simulink model "gm_uz_JL_pmsmModel"  (R2025a)
settings: Solver=FixedStepDiscrete  StartTime=0.0  StopTime=1  RelTol=1e-3
libraries: hdlmdlgenlib x2
(part 1 of 2)
settings Model: Creator=jonat  LastModifiedBy=jonat
settings SolverCC: AlgebraicLoopSolver=TrustRegion
settings DataIOCC: LimitDataPoints=on  SaveOutput=off  SaveTime=off
settings OptimizationCC: BlockReduction=off  ConditionallyExecuteInputs=off  DefaultParameterBehavior=Inlined  InheritOutputTypeSmallerThanSingle=on  DefaultUnderspecifiedDataType=single  LifeSpan=inf
settings DebuggingCC: AlgebraicLoopMsg=error  InheritedTsInSrcMsg=none  SingleTaskRateTransMsg=error  SignalLabelMismatchMsg=warning  UnconnectedInputMsg=warning  UnconnectedOutputMsg=warning  UnconnectedLineMsg=warning  AllowSymbolicDim=off  ModelReferenceVersionMismatchMessage=warning  ModelReferenceIOMismatchMessage=warning  ModelReferenceNoExplicitFinalValueMsg=warning  StrictBusMsg=ErrorOnBusTreatedAsVector  BusNameAdapt=ErrorWithoutRepair  SFUnexpectedBacktrackingDiag=warning  SFNoUnconditionalDefaultTransitionDiag=warning  SFExecutionAtInitializationDiag=none  ArithmeticOperatorsInVariantConditions=warning
settings HardwareCC: ProdBitPerPointer=32.0  ProdBitPerSizeT=32.0  ProdBitPerPtrDiffT=32.0  ProdLargestAtomicFloat=None  ProdIntDivRoundTo=Undefined  ProdEndianess=Unspecified  ProdWordSize=32.0  ProdHWDeviceType=ASIC/FPGA->ASIC/FPGA  TargetBitPerPointer=64.0  TargetBitPerSizeT=64.0  TargetBitPerPtrDiffT=64.0  TargetLongLongMode=on  TargetIntDivRoundTo=Zero  TargetEndianess=LittleEndian  TargetWordSize=64.0  TargetHWDeviceType=Custom Processor->MATLAB Host Computer  ProdEqTarget=off
settings ModelReferenceCC: EnableRefExpFcnMdlSchedulingChecks=on
settings SFSimCC: SimUseLocalCustomCode=off  CustomCodeUndefinedFunction=UseInterfaceOnly
settings RTWCC: RTWUseLocalCustomCode=off  GPUComputeCapability=3.5
settings CodeAppCC: StateflowObjectComments=on
settings GRTTargetCC: TargetLangStandard=C89/C90 (ANSI)
settings ConfigComp: CovScope=ReferencedModels  CovMetricSettings=dw  CovSaveCumulativeToWorkspaceVar=on  CovSaveSingleToWorkspaceVar=on  CovExternalEMLEnable=off  CovSFcnEnable=off

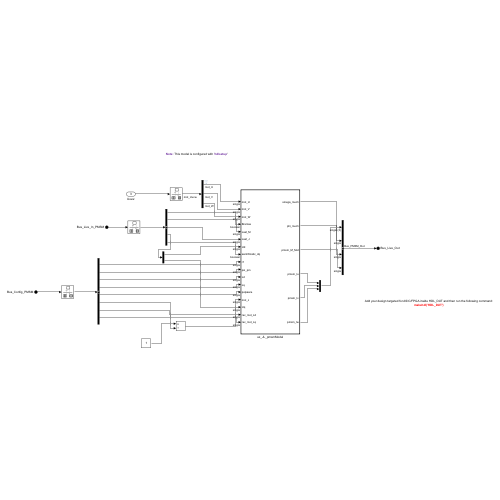
[thumbnail: Simulink's stored preview of the top-level diagram]
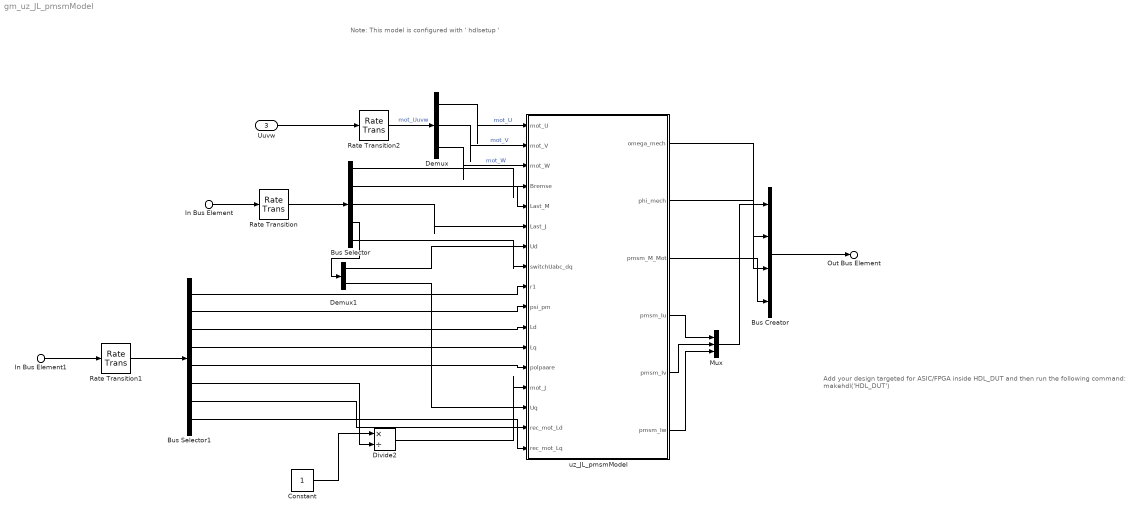
== system gm_uz_JL_pmsmModel ==
  note: Add your design targeted for ASIC/FPGA inside HDL_DUT and then run the following command:
      | makehdl('HDL_DUT')
  note: Note: This model is configured with ' hdlsetup '
  In Bus Element : Inport  PortName=Bus_Live_In_PMSM
  In Bus Element1 : Inport  Port=2  PortName=Bus_Config_PMSM
  Uuvw : Inport  Port=3
  Bus Creator : BusCreator  Inputs=4  OutDataTypeStr=Bus: Bus_PMSM_Out  NonVirtualBus=on
      settings: InheritFromInputs=off
  Bus Selector : BusSelector  OutputSignals=Bremse,Last_M,Last_J,Udq,switchUabc_dq
  Bus Selector1 : BusSelector  OutputSignals=mot_R1,mot_psi_pm,mot_Ld,mot_Lq,mot_p,mot_J,rec_mot_Ld,rec_mot_Lq
  Constant : Constant
  Demux : Demux  Outputs=3
  Demux1 : Demux  Outputs=2
  Divide2 : Product  Inputs=*/  OutDataTypeStr=single
  Mux : Mux  Inputs=3
  Rate Transition : RateTransition  OutPortSampleTime=1/5e5
  Rate Transition1 : RateTransition  OutPortSampleTime=1/5e5
  Rate Transition2 : RateTransition  OutPortSampleTime=1/5e5
  uz_JL_pmsmModel : Subsystem  TreatAsAtomicUnit=on
  Out Bus Element : Outport  PortName=Bus_Live_Out
  wires:
  Bus Selector1/8 -> uz_JL_pmsmModel/17(rec_mot_Lq)
  Bus Selector1/7 -> uz_JL_pmsmModel/16(rec_mot_Ld)
  Demux1/2 -> uz_JL_pmsmModel/15(Uq)
  Demux1/1 -> uz_JL_pmsmModel/7(Ud)
  Mux/1 -> Bus Creator/1
  uz_JL_pmsmModel/6(pmsm_Iw) -> Mux/3
  uz_JL_pmsmModel/5(pmsm_Iv) -> Mux/2
  uz_JL_pmsmModel/4(pmsm_Iu) -> Mux/1
  Demux/1 -> uz_JL_pmsmModel/1(mot_U)  "mot_U"
  Rate Transition2/1 -> Demux/1  "mot_Uuvw"
  Demux/2 -> uz_JL_pmsmModel/2(mot_V)  "mot_V"
  Demux/3 -> uz_JL_pmsmModel/3(mot_W)  "mot_W"
  Divide2/1 -> uz_JL_pmsmModel/14(mot_J)
  Constant/1 -> Divide2/1
  uz_JL_pmsmModel/3(pmsm_M_Mot) -> Bus Creator/4
  uz_JL_pmsmModel/2(phi_mech) -> Bus Creator/3
  uz_JL_pmsmModel/1(omega_mech) -> Bus Creator/2
  Bus Selector1/6 -> Divide2/2
  Bus Selector1/5 -> uz_JL_pmsmModel/13(polpaare)
  Bus Selector1/4 -> uz_JL_pmsmModel/12(Lq)
  Bus Selector1/3 -> uz_JL_pmsmModel/11(Ld)
  Bus Selector1/2 -> uz_JL_pmsmModel/10(psi_pm)
  Bus Selector1/1 -> uz_JL_pmsmModel/9(r1)
  Bus Selector/5 -> uz_JL_pmsmModel/8(switchUabc_dq)
  Bus Selector/4 -> Demux1/1
  Bus Selector/3 -> uz_JL_pmsmModel/6(Last_J)
  Bus Selector/2 -> uz_JL_pmsmModel/5(Last_M)
  Bus Selector/1 -> uz_JL_pmsmModel/4(Bremse)
  Uuvw/1 -> Rate Transition2/1
  Rate Transition1/1 -> Bus Selector1/1
  Rate Transition/1 -> Bus Selector/1
  Bus Creator/1 -> Out Bus Element/1
  In Bus Element1/1 -> Rate Transition1/1
  In Bus Element/1 -> Rate Transition/1

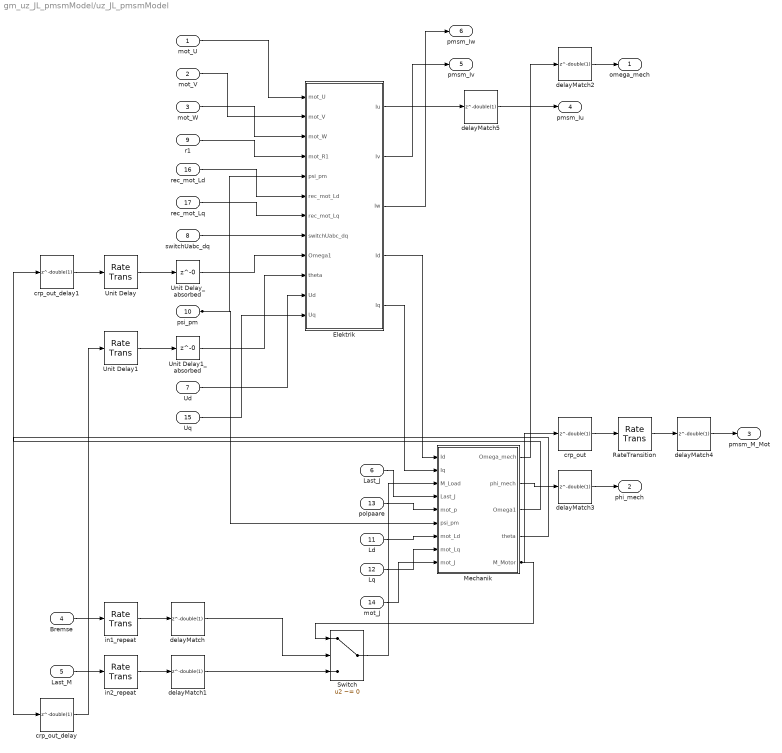
== system gm_uz_JL_pmsmModel/uz_JL_pmsmModel ==
  mot_U : Inport  OutDataTypeStr=single  PortDimensions=1  SampleTime=2e-06
  mot_V : Inport  Port=2  OutDataTypeStr=single  PortDimensions=1  SampleTime=2e-06
  mot_W : Inport  Port=3  OutDataTypeStr=single  PortDimensions=1  SampleTime=2e-06
  Bremse : Inport  Port=4  OutDataTypeStr=boolean  PortDimensions=1  SampleTime=2e-06
  Last_M : Inport  Port=5  OutDataTypeStr=single  PortDimensions=1  SampleTime=2e-06
  Last_J : Inport  Port=6  OutDataTypeStr=single  PortDimensions=1  SampleTime=2e-06
  Ud : Inport  Port=7  OutDataTypeStr=single  PortDimensions=1  SampleTime=2e-06
  switchUabc_dq : Inport  Port=8  OutDataTypeStr=boolean  PortDimensions=1  SampleTime=2e-06
  r1 : Inport  Port=9  OutDataTypeStr=single  PortDimensions=1  SampleTime=2e-06
  psi_pm : Inport  Port=10  OutDataTypeStr=single  PortDimensions=1  SampleTime=2e-06
  Ld : Inport  Port=11  OutDataTypeStr=single  PortDimensions=1  SampleTime=2e-06
  Lq : Inport  Port=12  OutDataTypeStr=single  PortDimensions=1  SampleTime=2e-06
  polpaare : Inport  Port=13  OutDataTypeStr=single  PortDimensions=1  SampleTime=2e-06
  mot_J : Inport  Port=14  OutDataTypeStr=single  PortDimensions=1  SampleTime=2e-06
  Uq : Inport  Port=15  OutDataTypeStr=single  PortDimensions=1  SampleTime=2e-06
  rec_mot_Ld : Inport  Port=16  OutDataTypeStr=single  PortDimensions=1  SampleTime=2e-06
  rec_mot_Lq : Inport  Port=17  OutDataTypeStr=single  PortDimensions=1  SampleTime=2e-06
  Elektrik : Subsystem
  Mechanik : Subsystem
  RateTransition : RateTransition  InitialCondition=double(0)  OutPortSampleTimeOpt=Multiple of input port sample time  OutPortSampleTimeMultiple=100
  Switch : Switch  Criteria=u2 ~= 0  Threshold="fi(0,0,1,0,\"hex\",\"0\")"  OutDataTypeStr=single  SampleTime=2e-08  SaturateOnIntegerOverflow=off  InputSameDT=off
  Unit Delay : RateTransition  InitialCondition=double(0)  OutPortSampleTimeOpt=Multiple of input port sample time  OutPortSampleTimeMultiple=100
  Unit Delay1 : RateTransition  InitialCondition=double(0)  OutPortSampleTimeOpt=Multiple of input port sample time  OutPortSampleTimeMultiple=100
  Unit Delay1_absorbed : Delay  DelayLength=0
  Unit Delay_absorbed : Delay  DelayLength=0
  crp_out : Delay  DelayLength=double(1)  InitialCondition=0  SampleTime=2e-08
  crp_out_delay : Delay  DelayLength=double(1)  InitialCondition=0  SampleTime=2e-08
  crp_out_delay1 : Delay  DelayLength=double(1)  InitialCondition=0  SampleTime=2e-08
  delayMatch : Delay  DelayLength=double(1)  InitialCondition=0  SampleTime=2e-08
  delayMatch1 : Delay  DelayLength=double(1)  InitialCondition=0  SampleTime=2e-08
  delayMatch{2..5} (4 alike) : Delay  DelayLength=double(1)  InitialCondition=0  SampleTime=2e-06
  in1_repeat : RateTransition  Integrity=off  Deterministic=off  OutPortSampleTimeOpt=Multiple of input port sample time  OutPortSampleTimeMultiple=1/100
  in2_repeat : RateTransition  Integrity=off  Deterministic=off  OutPortSampleTimeOpt=Multiple of input port sample time  OutPortSampleTimeMultiple=1/100
  omega_mech : Outport  SampleTime=2e-06
  phi_mech : Outport  Port=2  SampleTime=2e-06
  pmsm_M_Mot : Outport  Port=3  SampleTime=2e-06
  pmsm_Iu : Outport  Port=4  SampleTime=2e-06
  pmsm_Iv : Outport  Port=5  SampleTime=2e-06
  pmsm_Iw : Outport  Port=6  SampleTime=2e-06
  wires:
  in2_repeat/1 -> delayMatch1/1
  crp_out_delay1/1 -> Unit Delay/1
  Unit Delay/1 -> Unit Delay_absorbed/1
  Ud/1 -> Elektrik/11(Ud)
  Bremse/1 -> in1_repeat/1
  Unit Delay1/1 -> Unit Delay1_absorbed/1
  Last_M/1 -> in2_repeat/1
  crp_out_delay/1 -> Unit Delay1/1
  in1_repeat/1 -> delayMatch/1
  Elektrik/2(Iv) -> pmsm_Iv/1
  mot_U/1 -> Elektrik/1(mot_U)
  polpaare/1 -> Mechanik/5(mot_p)
  mot_V/1 -> Elektrik/2(mot_V)
  delayMatch/1 -> Switch/2
  mot_W/1 -> Elektrik/3(mot_W)
  delayMatch4/1 -> pmsm_M_Mot/1
  r1/1 -> Elektrik/4(mot_R1)
  Elektrik/5(Iq) -> Mechanik/2(Iq)
  rec_mot_Ld/1 -> Elektrik/6(rec_mot_Ld)
  rec_mot_Lq/1 -> Elektrik/7(rec_mot_Lq)
  Mechanik/3(Omega1) -> crp_out_delay1/1
  switchUabc_dq/1 -> Elektrik/8(switchUabc_dq)
  Unit Delay_absorbed/1 -> Elektrik/9(Omega1)
  psi_pm/1 -> Mechanik/6(psi_pm), Elektrik/5(psi_pm)
  Switch/1 -> Mechanik/3(M_Load)
  Unit Delay1_absorbed/1 -> Elektrik/10(theta)
  Uq/1 -> Elektrik/12(Uq)
  Ld/1 -> Mechanik/7(mot_Ld)
  Elektrik/4(Id) -> Mechanik/1(Id)
  delayMatch1/1 -> Switch/3
  Elektrik/1(Iu) -> delayMatch5/1
  Elektrik/3(Iw) -> pmsm_Iw/1
  Last_J/1 -> Mechanik/4(Last_J)
  Lq/1 -> Mechanik/8(mot_Lq)
  delayMatch3/1 -> phi_mech/1
  mot_J/1 -> Mechanik/9(mot_J)
  delayMatch5/1 -> pmsm_Iu/1
  Mechanik/1(Omega_mech) -> delayMatch2/1
  Mechanik/2(phi_mech) -> delayMatch3/1
  Mechanik/4(theta) -> crp_out_delay/1
  Mechanik/5(M_Motor) -> crp_out/1, Switch/1
  delayMatch2/1 -> omega_mech/1
  crp_out/1 -> RateTransition/1
  RateTransition/1 -> delayMatch4/1

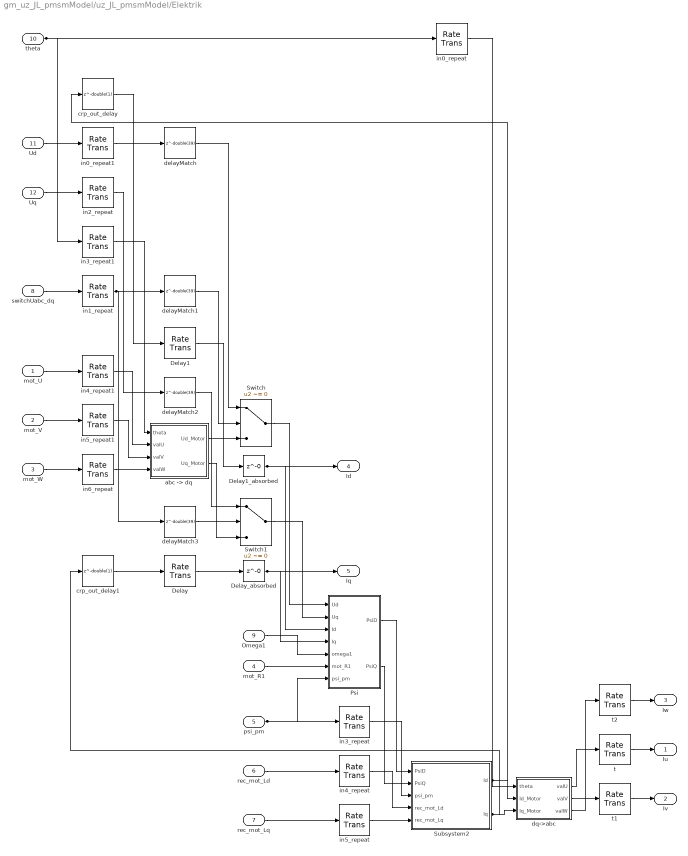
== system gm_uz_JL_pmsmModel/uz_JL_pmsmModel/Elektrik ==
  mot_U : Inport  OutDataTypeStr=single  PortDimensions=1  SampleTime=2e-06
  mot_V : Inport  Port=2  OutDataTypeStr=single  PortDimensions=1  SampleTime=2e-06
  mot_W : Inport  Port=3  OutDataTypeStr=single  PortDimensions=1  SampleTime=2e-06
  mot_R1 : Inport  Port=4  OutDataTypeStr=single  PortDimensions=1  SampleTime=2e-06
  psi_pm : Inport  Port=5  OutDataTypeStr=single  PortDimensions=1  SampleTime=2e-06
  rec_mot_Ld : Inport  Port=6  OutDataTypeStr=single  PortDimensions=1  SampleTime=2e-06
  rec_mot_Lq : Inport  Port=7  OutDataTypeStr=single  PortDimensions=1  SampleTime=2e-06
  switchUabc_dq : Inport  Port=8  OutDataTypeStr=boolean  PortDimensions=1  SampleTime=2e-06
  Omega1 : Inport  Port=9  OutDataTypeStr=single  PortDimensions=1  SampleTime=2e-06
  theta : Inport  Port=10  OutDataTypeStr=single  PortDimensions=1  SampleTime=2e-06
  Ud : Inport  Port=11  OutDataTypeStr=single  PortDimensions=1  SampleTime=2e-06
  Uq : Inport  Port=12  OutDataTypeStr=single  PortDimensions=1  SampleTime=2e-06
  Delay : RateTransition  InitialCondition=double(0)  OutPortSampleTimeOpt=Multiple of input port sample time  OutPortSampleTimeMultiple=100
  Delay1 : RateTransition  InitialCondition=double(0)  OutPortSampleTimeOpt=Multiple of input port sample time  OutPortSampleTimeMultiple=100
  Delay1_absorbed : Delay  DelayLength=0
  Delay_absorbed : Delay  DelayLength=0
  Psi : Subsystem
  Subsystem2 : Subsystem
  Switch : Switch  Criteria=u2 ~= 0  Threshold="fi(0,0,1,0,\"hex\",\"0\")"  OutDataTypeStr=single  SampleTime=2e-08  SaturateOnIntegerOverflow=off  InputSameDT=off
  Switch1 : Switch  Criteria=u2 ~= 0  Threshold="fi(0,0,1,0,\"hex\",\"0\")"  OutDataTypeStr=single  SampleTime=2e-08  SaturateOnIntegerOverflow=off  InputSameDT=off
  "abc -> dq" : Subsystem
  crp_out_delay : Delay  DelayLength=double(1)  InitialCondition=0  SampleTime=2e-08
  crp_out_delay1 : Delay  DelayLength=double(1)  InitialCondition=0  SampleTime=2e-08
  delayMatch{,1..3} (4 alike) : Delay  DelayLength=double(39)  InitialCondition=0  SampleTime=2e-08
  dq->abc : Subsystem
  in0_repeat : RateTransition  Integrity=off  Deterministic=off  OutPortSampleTimeOpt=Multiple of input port sample time  OutPortSampleTimeMultiple=1/100
  in0_repeat1 : RateTransition  Integrity=off  Deterministic=off  OutPortSampleTimeOpt=Multiple of input port sample time  OutPortSampleTimeMultiple=1/100
  in1_repeat : RateTransition  Integrity=off  Deterministic=off  OutPortSampleTimeOpt=Multiple of input port sample time  OutPortSampleTimeMultiple=1/100
  in2_repeat : RateTransition  Integrity=off  Deterministic=off  OutPortSampleTimeOpt=Multiple of input port sample time  OutPortSampleTimeMultiple=1/100
  in3_repeat : RateTransition  Integrity=off  Deterministic=off  OutPortSampleTimeOpt=Multiple of input port sample time  OutPortSampleTimeMultiple=1/100
  in3_repeat1 : RateTransition  Integrity=off  Deterministic=off  OutPortSampleTimeOpt=Multiple of input port sample time  OutPortSampleTimeMultiple=1/100
  in4_repeat : RateTransition  Integrity=off  Deterministic=off  OutPortSampleTimeOpt=Multiple of input port sample time  OutPortSampleTimeMultiple=1/100
  in4_repeat1 : RateTransition  Integrity=off  Deterministic=off  OutPortSampleTimeOpt=Multiple of input port sample time  OutPortSampleTimeMultiple=1/100
  in5_repeat : RateTransition  Integrity=off  Deterministic=off  OutPortSampleTimeOpt=Multiple of input port sample time  OutPortSampleTimeMultiple=1/100
  in5_repeat1 : RateTransition  Integrity=off  Deterministic=off  OutPortSampleTimeOpt=Multiple of input port sample time  OutPortSampleTimeMultiple=1/100
  in6_repeat : RateTransition  Integrity=off  Deterministic=off  OutPortSampleTimeOpt=Multiple of input port sample time  OutPortSampleTimeMultiple=1/100
  t : RateTransition  InitialCondition=double(0)  OutPortSampleTimeOpt=Multiple of input port sample time  OutPortSampleTimeMultiple=100
  t1 : RateTransition  InitialCondition=double(0)  OutPortSampleTimeOpt=Multiple of input port sample time  OutPortSampleTimeMultiple=100
  t2 : RateTransition  InitialCondition=double(0)  OutPortSampleTimeOpt=Multiple of input port sample time  OutPortSampleTimeMultiple=100
  Iu : Outport  SampleTime=2e-06
  Iv : Outport  Port=2  SampleTime=2e-06
  Iw : Outport  Port=3  SampleTime=2e-06
  Id : Outport  Port=4  SampleTime=2e-06
  Iq : Outport  Port=5  SampleTime=2e-06
  wires:
  theta/1 -> in0_repeat/1, in3_repeat1/1
  mot_V/1 -> in5_repeat1/1
  mot_U/1 -> in4_repeat1/1
  mot_W/1 -> in6_repeat/1
  Ud/1 -> in0_repeat1/1
  Uq/1 -> in2_repeat/1
  switchUabc_dq/1 -> in1_repeat/1
  Switch1/1 -> Psi/2(Uq)
  crp_out_delay/1 -> Delay1/1
  in5_repeat1/1 -> "abc -> dq"/3(valV)
  in0_repeat1/1 -> delayMatch/1
  in2_repeat/1 -> delayMatch2/1
  t1/1 -> Iv/1
  in6_repeat/1 -> "abc -> dq"/4(valW)
  in3_repeat1/1 -> "abc -> dq"/1(theta)
  in1_repeat/1 -> delayMatch3/1, delayMatch1/1
  t/1 -> Iu/1
  in4_repeat1/1 -> "abc -> dq"/2(valU)
  crp_out_delay1/1 -> Delay/1
  delayMatch/1 -> Switch/1
  dq->abc/2(valV) -> t1/1
  "abc -> dq"/1(Ud_Motor) -> Switch/3
  delayMatch1/1 -> Switch/2
  Subsystem2/2(Iq) -> crp_out_delay1/1, dq->abc/3(Iq_Motor)
  Delay1/1 -> Delay1_absorbed/1
  delayMatch2/1 -> Switch1/1
  "abc -> dq"/2(Uq_Motor) -> Switch1/3
  delayMatch3/1 -> Switch1/2
  Delay/1 -> Delay_absorbed/1
  Subsystem2/1(Id) -> crp_out_delay/1, dq->abc/2(Id_Motor)
  rec_mot_Ld/1 -> in4_repeat/1
  Switch/1 -> Psi/1(Ud)
  Delay1_absorbed/1 -> Id/1, Psi/3(Id)
  Delay_absorbed/1 -> Iq/1, Psi/4(Iq)
  Omega1/1 -> Psi/5(omega1)
  mot_R1/1 -> Psi/6(mot_R1)
  psi_pm/1 -> in3_repeat/1, Psi/7(psi_pm)
  in4_repeat/1 -> Subsystem2/4(rec_mot_Ld)
  rec_mot_Lq/1 -> in5_repeat/1
  dq->abc/1(valU) -> t/1
  Psi/1(PsiD) -> Subsystem2/1(PsiD)
  Psi/2(PsiQ) -> Subsystem2/2(PsiQ)
  in3_repeat/1 -> Subsystem2/3(psi_pm)
  in5_repeat/1 -> Subsystem2/5(rec_mot_Lq)
  in0_repeat/1 -> dq->abc/1(theta)
  dq->abc/3(valW) -> t2/1
  t2/1 -> Iw/1

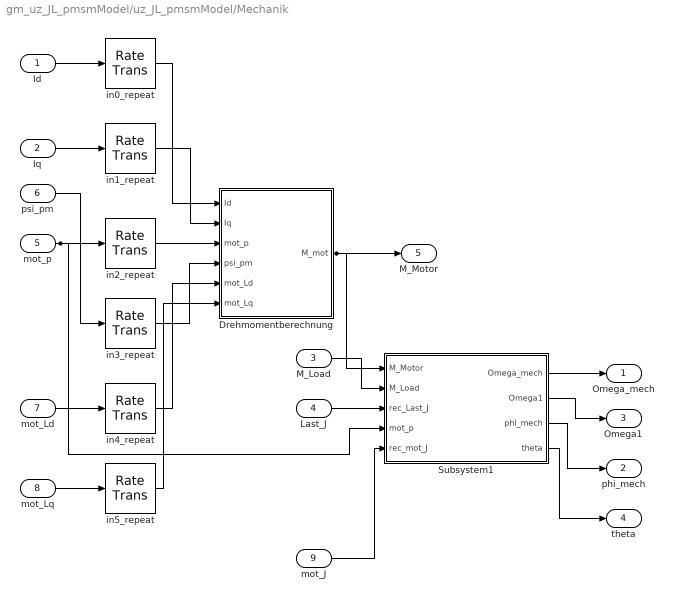
== system gm_uz_JL_pmsmModel/uz_JL_pmsmModel/Mechanik ==
  Id : Inport  OutDataTypeStr=single  PortDimensions=1  SampleTime=2e-06
  Iq : Inport  Port=2  OutDataTypeStr=single  PortDimensions=1  SampleTime=2e-06
  M_Load : Inport  Port=3  OutDataTypeStr=single  PortDimensions=1  SampleTime=2e-08
  Last_J : Inport  Port=4  OutDataTypeStr=single  PortDimensions=1  SampleTime=2e-06
  mot_p : Inport  Port=5  OutDataTypeStr=single  PortDimensions=1  SampleTime=2e-06
  psi_pm : Inport  Port=6  OutDataTypeStr=single  PortDimensions=1  SampleTime=2e-06
  mot_Ld : Inport  Port=7  OutDataTypeStr=single  PortDimensions=1  SampleTime=2e-06
  mot_Lq : Inport  Port=8  OutDataTypeStr=single  PortDimensions=1  SampleTime=2e-06
  mot_J : Inport  Port=9  OutDataTypeStr=single  PortDimensions=1  SampleTime=2e-06
  Drehmomentberechnung : Subsystem
  Subsystem1 : Subsystem
  in0_repeat : RateTransition  Integrity=off  Deterministic=off  OutPortSampleTimeOpt=Multiple of input port sample time  OutPortSampleTimeMultiple=1/100
  in1_repeat : RateTransition  Integrity=off  Deterministic=off  OutPortSampleTimeOpt=Multiple of input port sample time  OutPortSampleTimeMultiple=1/100
  in2_repeat : RateTransition  Integrity=off  Deterministic=off  OutPortSampleTimeOpt=Multiple of input port sample time  OutPortSampleTimeMultiple=1/100
  in3_repeat : RateTransition  Integrity=off  Deterministic=off  OutPortSampleTimeOpt=Multiple of input port sample time  OutPortSampleTimeMultiple=1/100
  in4_repeat : RateTransition  Integrity=off  Deterministic=off  OutPortSampleTimeOpt=Multiple of input port sample time  OutPortSampleTimeMultiple=1/100
  in5_repeat : RateTransition  Integrity=off  Deterministic=off  OutPortSampleTimeOpt=Multiple of input port sample time  OutPortSampleTimeMultiple=1/100
  Omega_mech : Outport  SampleTime=2e-06
  phi_mech : Outport  Port=2  SampleTime=2e-06
  Omega1 : Outport  Port=3  SampleTime=2e-08
  theta : Outport  Port=4  SampleTime=2e-08
  M_Motor : Outport  Port=5  SampleTime=2e-08
  wires:
  mot_J/1 -> Subsystem1/5(rec_mot_J)
  in0_repeat/1 -> Drehmomentberechnung/1(Id)
  Id/1 -> in0_repeat/1
  Iq/1 -> in1_repeat/1
  psi_pm/1 -> in3_repeat/1
  mot_p/1 -> Subsystem1/4(mot_p), in2_repeat/1
  in4_repeat/1 -> Drehmomentberechnung/5(mot_Ld)
  mot_Ld/1 -> in4_repeat/1
  mot_Lq/1 -> in5_repeat/1
  Subsystem1/1(Omega_mech) -> Omega_mech/1
  in1_repeat/1 -> Drehmomentberechnung/2(Iq)
  in2_repeat/1 -> Drehmomentberechnung/3(mot_p)
  in3_repeat/1 -> Drehmomentberechnung/4(psi_pm)
  in5_repeat/1 -> Drehmomentberechnung/6(mot_Lq)
  Subsystem1/3(phi_mech) -> phi_mech/1
  Drehmomentberechnung/1(M_mot) -> M_Motor/1, Subsystem1/1(M_Motor)
  M_Load/1 -> Subsystem1/2(M_Load)
  Subsystem1/2(Omega1) -> Omega1/1
  Last_J/1 -> Subsystem1/3(rec_Last_J)
  Subsystem1/4(theta) -> theta/1

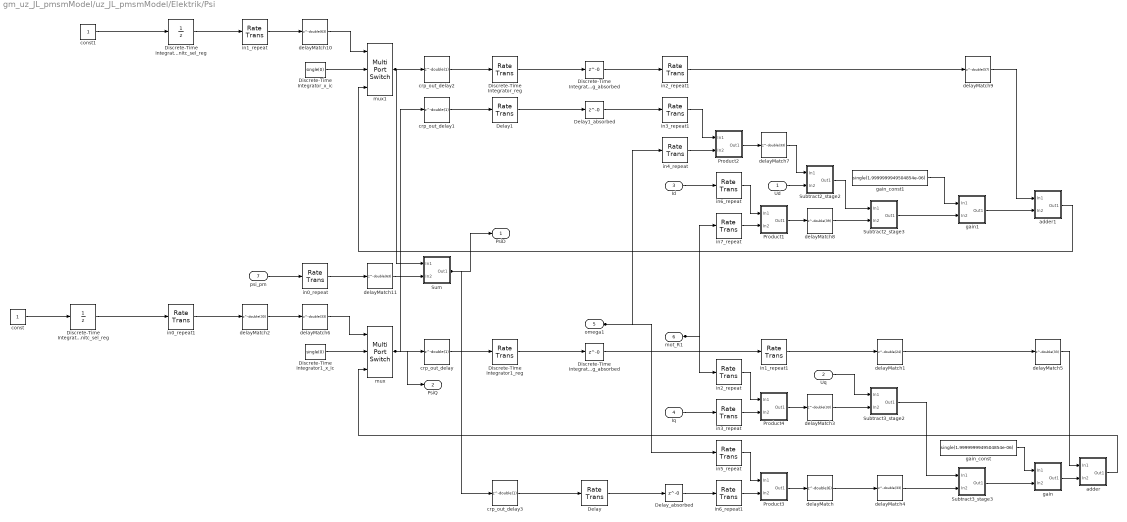
== system gm_uz_JL_pmsmModel/uz_JL_pmsmModel/Elektrik/Psi ==
  Ud : Inport  OutDataTypeStr=single  PortDimensions=1  SampleTime=2e-08
  Uq : Inport  Port=2  OutDataTypeStr=single  PortDimensions=1  SampleTime=2e-08
  Id : Inport  Port=3  OutDataTypeStr=single  PortDimensions=1  SampleTime=2e-06
  Iq : Inport  Port=4  OutDataTypeStr=single  PortDimensions=1  SampleTime=2e-06
  omega1 : Inport  Port=5  OutDataTypeStr=single  PortDimensions=1  SampleTime=2e-06
  mot_R1 : Inport  Port=6  OutDataTypeStr=single  PortDimensions=1  SampleTime=2e-06
  psi_pm : Inport  Port=7  OutDataTypeStr=single  PortDimensions=1  SampleTime=2e-06
  Delay : RateTransition  InitialCondition=double(0)  OutPortSampleTimeOpt=Multiple of input port sample time  OutPortSampleTimeMultiple=100
  Delay1 : RateTransition  InitialCondition=double(0)  OutPortSampleTimeOpt=Multiple of input port sample time  OutPortSampleTimeMultiple=100
  Delay1_absorbed : Delay  DelayLength=0
  Delay_absorbed : Delay  DelayLength=0
  Discrete-Time Integrator1_initc_sel_reg : UnitDelay  InitialCondition=double(0)  SampleTime=2e-06
  Discrete-Time Integrator1_reg : RateTransition  InitialCondition=double(0)  OutPortSampleTimeOpt=Multiple of input port sample time  OutPortSampleTimeMultiple=100
  Discrete-Time Integrator1_reg_absorbed : Delay  DelayLength=0
  Discrete-Time Integrator1_x_ic : Constant  Value=single(0)  OutDataTypeStr=single  SampleTime=2e-08
  Discrete-Time Integrator_initc_sel_reg : UnitDelay  InitialCondition=double(0)  SampleTime=2e-06
  Discrete-Time Integrator_reg : RateTransition  InitialCondition=double(0)  OutPortSampleTimeOpt=Multiple of input port sample time  OutPortSampleTimeMultiple=100
  Discrete-Time Integrator_reg_absorbed : Delay  DelayLength=0
  Discrete-Time Integrator_x_ic : Constant  Value=single(0)  OutDataTypeStr=single  SampleTime=2e-08
  Product1 : Subsystem
      mask Display: disp('NFP\nmul');
  Product2 : Subsystem
      mask Display: disp('NFP\nmul');
  Product3 : Subsystem
      mask Display: disp('NFP\nmul');
  Product4 : Subsystem
      mask Display: disp('NFP\nmul');
  Subtract2_stage2 : Subsystem
      mask Display: disp('NFP\nadd');
  Subtract2_stage3 : Subsystem
      mask Display: disp('NFP\nadd');
  Subtract3_stage2 : Subsystem
      mask Display: disp('NFP\nadd');
  Subtract3_stage3 : Subsystem
      mask Display: disp('NFP\nadd');
  Sum : Subsystem
      mask Display: disp('NFP\nadd');
  adder : Subsystem
      mask Display: disp('NFP\nadd');
  adder1 : Subsystem
      mask Display: disp('NFP\nadd');
  const : Constant  OutDataTypeStr=fixdt(0, 1, 0)  SampleTime=2e-06
  const1 : Constant  OutDataTypeStr=fixdt(0, 1, 0)  SampleTime=2e-06
  crp_out_delay{,1..3} (4 alike) : Delay  DelayLength=double(1)  InitialCondition=0  SampleTime=2e-08
  delayMatch : Delay  DelayLength=double(6)  InitialCondition=0  SampleTime=2e-08
  delayMatch1 : Delay  DelayLength=double(24)  InitialCondition=0  SampleTime=2e-08
  delayMatch10 : Delay  DelayLength=double(63)  InitialCondition=0  SampleTime=2e-08
  delayMatch11 : Delay  DelayLength=double(63)  InitialCondition=0  SampleTime=2e-08
  delayMatch2 : Delay  DelayLength=double(30)  InitialCondition=0  SampleTime=2e-08
  delayMatch{3..7} (5 alike) : Delay  DelayLength=double(33)  InitialCondition=0  SampleTime=2e-08
  delayMatch8 : Delay  DelayLength=double(39)  InitialCondition=0  SampleTime=2e-08
  delayMatch9 : Delay  DelayLength=double(57)  InitialCondition=0  SampleTime=2e-08
  gain : Subsystem
      mask Display: disp('NFP\nmul');
  gain1 : Subsystem
      mask Display: disp('NFP\nmul');
  gain_const : Constant  Value=single(1.9999999949504854e-06)  OutDataTypeStr=single  SampleTime=2e-08
  gain_const1 : Constant  Value=single(1.9999999949504854e-06)  OutDataTypeStr=single  SampleTime=2e-08
  in0_repeat : RateTransition  Integrity=off  Deterministic=off  OutPortSampleTimeOpt=Multiple of input port sample time  OutPortSampleTimeMultiple=1/100
  in0_repeat1 : RateTransition  Integrity=off  Deterministic=off  OutPortSampleTimeOpt=Multiple of input port sample time  OutPortSampleTimeMultiple=1/100
  in1_repeat : RateTransition  Integrity=off  Deterministic=off  OutPortSampleTimeOpt=Multiple of input port sample time  OutPortSampleTimeMultiple=1/100
  in1_repeat1 : RateTransition  Integrity=off  Deterministic=off  OutPortSampleTimeOpt=Multiple of input port sample time  OutPortSampleTimeMultiple=1/100
  in2_repeat : RateTransition  Integrity=off  Deterministic=off  OutPortSampleTimeOpt=Multiple of input port sample time  OutPortSampleTimeMultiple=1/100
  in2_repeat1 : RateTransition  Integrity=off  Deterministic=off  OutPortSampleTimeOpt=Multiple of input port sample time  OutPortSampleTimeMultiple=1/100
  in3_repeat : RateTransition  Integrity=off  Deterministic=off  OutPortSampleTimeOpt=Multiple of input port sample time  OutPortSampleTimeMultiple=1/100
  in3_repeat1 : RateTransition  Integrity=off  Deterministic=off  OutPortSampleTimeOpt=Multiple of input port sample time  OutPortSampleTimeMultiple=1/100
  in4_repeat : RateTransition  Integrity=off  Deterministic=off  OutPortSampleTimeOpt=Multiple of input port sample time  OutPortSampleTimeMultiple=1/100
  in5_repeat : RateTransition  Integrity=off  Deterministic=off  OutPortSampleTimeOpt=Multiple of input port sample time  OutPortSampleTimeMultiple=1/100
  in6_repeat : RateTransition  Integrity=off  Deterministic=off  OutPortSampleTimeOpt=Multiple of input port sample time  OutPortSampleTimeMultiple=1/100
  in6_repeat1 : RateTransition  Integrity=off  Deterministic=off  OutPortSampleTimeOpt=Multiple of input port sample time  OutPortSampleTimeMultiple=1/100
  in7_repeat : RateTransition  Integrity=off  Deterministic=off  OutPortSampleTimeOpt=Multiple of input port sample time  OutPortSampleTimeMultiple=1/100
  mux : MultiPortSwitch  DataPortOrder=Zero-based contiguous  Inputs=2  DiagnosticForDefault=None  zeroidx=on  OutDataTypeStr=single  SampleTime=2e-08  SaturateOnIntegerOverflow=off  InputSameDT=off
  mux1 : MultiPortSwitch  DataPortOrder=Zero-based contiguous  Inputs=2  DiagnosticForDefault=None  zeroidx=on  OutDataTypeStr=single  SampleTime=2e-08  SaturateOnIntegerOverflow=off  InputSameDT=off
  PsiD : Outport  SampleTime=2e-08
  PsiQ : Outport  Port=2  SampleTime=2e-08
  wires:
  Discrete-Time Integrator_initc_sel_reg/1 -> in1_repeat/1
  const/1 -> Discrete-Time Integrator1_initc_sel_reg/1
  mux1/1 -> Sum/1(In1), crp_out_delay2/1
  Product4/1(Out1) -> delayMatch3/1
  const1/1 -> Discrete-Time Integrator_initc_sel_reg/1
  Product3/1(Out1) -> delayMatch/1
  in0_repeat1/1 -> delayMatch2/1
  Discrete-Time Integrator1_initc_sel_reg/1 -> in0_repeat1/1
  delayMatch3/1 -> Subtract3_stage2/2(In2)
  in1_repeat/1 -> delayMatch10/1
  delayMatch7/1 -> Subtract2_stage2/1(In1)
  delayMatch2/1 -> delayMatch6/1
  Discrete-Time Integrator1_x_ic/1 -> mux/2
  psi_pm/1 -> in0_repeat/1
  delayMatch10/1 -> mux1/1
  Discrete-Time Integrator_x_ic/1 -> mux1/2
  in0_repeat/1 -> delayMatch11/1
  Sum/1(Out1) -> PsiD/1, crp_out_delay3/1
  delayMatch9/1 -> adder1/1(In1)
  delayMatch6/1 -> mux/1
  delayMatch/1 -> delayMatch4/1
  delayMatch11/1 -> Sum/2(In2)
  crp_out_delay1/1 -> Delay1/1
  mux/1 -> PsiQ/1, crp_out_delay/1, crp_out_delay1/1
  crp_out_delay2/1 -> Discrete-Time Integrator_reg/1
  crp_out_delay/1 -> Discrete-Time Integrator1_reg/1
  omega1/1 -> in5_repeat/1, in4_repeat/1
  Discrete-Time Integrator_reg/1 -> Discrete-Time Integrator_reg_absorbed/1
  Delay1/1 -> Delay1_absorbed/1
  Discrete-Time Integrator1_reg/1 -> Discrete-Time Integrator1_reg_absorbed/1
  crp_out_delay3/1 -> Delay/1
  Iq/1 -> in3_repeat/1
  Product2/1(Out1) -> delayMatch7/1
  Discrete-Time Integrator_reg_absorbed/1 -> in2_repeat1/1
  delayMatch4/1 -> Subtract3_stage3/2(In2)
  delayMatch8/1 -> Subtract2_stage3/2(In2)
  Delay1_absorbed/1 -> in3_repeat1/1
  Delay/1 -> Delay_absorbed/1
  Discrete-Time Integrator1_reg_absorbed/1 -> in1_repeat1/1
  in2_repeat1/1 -> delayMatch9/1
  in1_repeat1/1 -> delayMatch1/1
  in3_repeat1/1 -> Product2/1(In1)
  Product1/1(Out1) -> delayMatch8/1
  in4_repeat/1 -> Product2/2(In2)
  Id/1 -> in6_repeat/1
  mot_R1/1 -> in2_repeat/1, in7_repeat/1
  Subtract3_stage3/1(Out1) -> gain/2(In2)
  Subtract3_stage2/1(Out1) -> Subtract3_stage3/1(In1)
  Delay_absorbed/1 -> in6_repeat1/1
  in6_repeat/1 -> Product1/1(In1)
  in7_repeat/1 -> Product1/2(In2)
  in2_repeat/1 -> Product4/1(In1)
  in3_repeat/1 -> Product4/2(In2)
  Subtract2_stage2/1(Out1) -> Subtract2_stage3/1(In1)
  in5_repeat/1 -> Product3/1(In1)
  in6_repeat1/1 -> Product3/2(In2)
  Ud/1 -> Subtract2_stage2/2(In2)
  Uq/1 -> Subtract3_stage2/1(In1)
  gain_const1/1 -> gain1/1(In1)
  Subtract2_stage3/1(Out1) -> gain1/2(In2)
  delayMatch1/1 -> delayMatch5/1
  gain1/1(Out1) -> adder1/2(In2)
  gain_const/1 -> gain/1(In1)
  adder1/1(Out1) -> mux1/3
  delayMatch5/1 -> adder/1(In1)
  gain/1(Out1) -> adder/2(In2)
  adder/1(Out1) -> mux/3

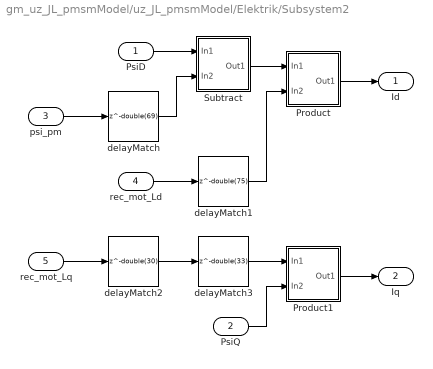
== system gm_uz_JL_pmsmModel/uz_JL_pmsmModel/Elektrik/Subsystem2 ==
  PsiD : Inport  OutDataTypeStr=single  PortDimensions=1  SampleTime=2e-08
  PsiQ : Inport  Port=2  OutDataTypeStr=single  PortDimensions=1  SampleTime=2e-08
  psi_pm : Inport  Port=3  OutDataTypeStr=single  PortDimensions=1  SampleTime=2e-08
  rec_mot_Ld : Inport  Port=4  OutDataTypeStr=single  PortDimensions=1  SampleTime=2e-08
  rec_mot_Lq : Inport  Port=5  OutDataTypeStr=single  PortDimensions=1  SampleTime=2e-08
  Product : Subsystem
      mask Display: disp('NFP\nmul');
  Product1 : Subsystem
      mask Display: disp('NFP\nmul');
  Subtract : Subsystem
      mask Display: disp('NFP\nadd');
  delayMatch : Delay  DelayLength=double(69)  InitialCondition=0  SampleTime=2e-08
  delayMatch1 : Delay  DelayLength=double(75)  InitialCondition=0  SampleTime=2e-08
  delayMatch2 : Delay  DelayLength=double(30)  InitialCondition=0  SampleTime=2e-08
  delayMatch3 : Delay  DelayLength=double(33)  InitialCondition=0  SampleTime=2e-08
  Id : Outport  SampleTime=2e-08
  Iq : Outport  Port=2  SampleTime=2e-08
  wires:
  psi_pm/1 -> delayMatch/1
  Subtract/1(Out1) -> Product/1(In1)
  delayMatch/1 -> Subtract/2(In2)
  rec_mot_Lq/1 -> delayMatch2/1
  PsiD/1 -> Subtract/1(In1)
  delayMatch1/1 -> Product/2(In2)
  rec_mot_Ld/1 -> delayMatch1/1
  delayMatch2/1 -> delayMatch3/1
  delayMatch3/1 -> Product1/1(In1)
  PsiQ/1 -> Product1/2(In2)
  Product/1(Out1) -> Id/1
  Product1/1(Out1) -> Iq/1

== system gm_uz_JL_pmsmModel/uz_JL_pmsmModel/Elektrik/abc -> dq ==
  theta : Inport  OutDataTypeStr=single  PortDimensions=1  SampleTime=2e-08
  valU : Inport  Port=2  OutDataTypeStr=single  PortDimensions=1  SampleTime=2e-08
  valV : Inport  Port=3  OutDataTypeStr=single  PortDimensions=1  SampleTime=2e-08
  valW : Inport  Port=4  OutDataTypeStr=single  PortDimensions=1  SampleTime=2e-08
  Clark Transformation : Subsystem
  Park-Transformation : Subsystem
  Ud_Motor : Outport  SampleTime=2e-08
  Uq_Motor : Outport  Port=2  SampleTime=2e-08
  wires:
  valU/1 -> Clark Transformation/1(valU)
  valV/1 -> Clark Transformation/2(valV)
  valW/1 -> Clark Transformation/3(valW)
  Park-Transformation/1(valD) -> Ud_Motor/1
  Clark Transformation/2(valBeta) -> Park-Transformation/3(valBeta)
  theta/1 -> Park-Transformation/1(theta)
  Park-Transformation/2(valQ) -> Uq_Motor/1
  Clark Transformation/1(valAlpha) -> Park-Transformation/2(valAlpha)

== system gm_uz_JL_pmsmModel/uz_JL_pmsmModel/Elektrik/dq->abc ==
  theta : Inport  OutDataTypeStr=single  PortDimensions=1  SampleTime=2e-08
  Id_Motor : Inport  Port=2  OutDataTypeStr=single  PortDimensions=1  SampleTime=2e-08
  Iq_Motor : Inport  Port=3  OutDataTypeStr=single  PortDimensions=1  SampleTime=2e-08
  Inverse Clarke-Transformation : Subsystem
  Inverse Park-Transformation : Subsystem
  valU : Outport  SampleTime=2e-08
  valV : Outport  Port=2  SampleTime=2e-08
  valW : Outport  Port=3  SampleTime=2e-08
  wires:
  Inverse Clarke-Transformation/3(valW) -> valW/1
  theta/1 -> Inverse Park-Transformation/1(theta)
  Inverse Clarke-Transformation/1(valU) -> valU/1
  Inverse Park-Transformation/2(valBeta) -> Inverse Clarke-Transformation/2(beta)
  Id_Motor/1 -> Inverse Park-Transformation/2(valD)
  Iq_Motor/1 -> Inverse Park-Transformation/3(valQ)
  Inverse Clarke-Transformation/2(valV) -> valV/1
  Inverse Park-Transformation/1(valAlpha) -> Inverse Clarke-Transformation/1(alpha)

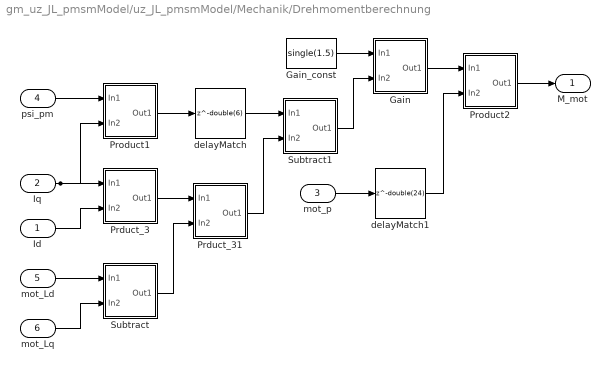
== system gm_uz_JL_pmsmModel/uz_JL_pmsmModel/Mechanik/Drehmomentberechnung ==
  Id : Inport  OutDataTypeStr=single  PortDimensions=1  SampleTime=2e-08
  Iq : Inport  Port=2  OutDataTypeStr=single  PortDimensions=1  SampleTime=2e-08
  mot_p : Inport  Port=3  OutDataTypeStr=single  PortDimensions=1  SampleTime=2e-08
  psi_pm : Inport  Port=4  OutDataTypeStr=single  PortDimensions=1  SampleTime=2e-08
  mot_Ld : Inport  Port=5  OutDataTypeStr=single  PortDimensions=1  SampleTime=2e-08
  mot_Lq : Inport  Port=6  OutDataTypeStr=single  PortDimensions=1  SampleTime=2e-08
  Gain : Subsystem
      mask Display: disp('NFP\nmul');
  Gain_const : Constant  Value=single(1.5)  OutDataTypeStr=single  SampleTime=2e-08
  Prduct_3 : Subsystem
      mask Display: disp('NFP\nmul');
  Prduct_31 : Subsystem
      mask Display: disp('NFP\nmul');
  Product1 : Subsystem
      mask Display: disp('NFP\nmul');
  Product2 : Subsystem
      mask Display: disp('NFP\nmul');
  Subtract : Subsystem
      mask Display: disp('NFP\nadd');
  Subtract1 : Subsystem
      mask Display: disp('NFP\nadd');
  delayMatch : Delay  DelayLength=double(6)  InitialCondition=0  SampleTime=2e-08
  delayMatch1 : Delay  DelayLength=double(24)  InitialCondition=0  SampleTime=2e-08
  M_mot : Outport  OutDataTypeStr=single  SampleTime=2e-08
  wires:
  Product1/1(Out1) -> delayMatch/1
  psi_pm/1 -> Product1/1(In1)
  Iq/1 -> Prduct_3/1(In1), Product1/2(In2)
  Id/1 -> Prduct_3/2(In2)
  mot_Ld/1 -> Subtract/1(In1)
  Prduct_3/1(Out1) -> Prduct_31/1(In1)
  mot_Lq/1 -> Subtract/2(In2)
  Subtract/1(Out1) -> Prduct_31/2(In2)
  delayMatch/1 -> Subtract1/1(In1)
  Prduct_31/1(Out1) -> Subtract1/2(In2)
  Gain_const/1 -> Gain/1(In1)
  Subtract1/1(Out1) -> Gain/2(In2)
  mot_p/1 -> delayMatch1/1
  Gain/1(Out1) -> Product2/1(In1)
  delayMatch1/1 -> Product2/2(In2)
  Product2/1(Out1) -> M_mot/1

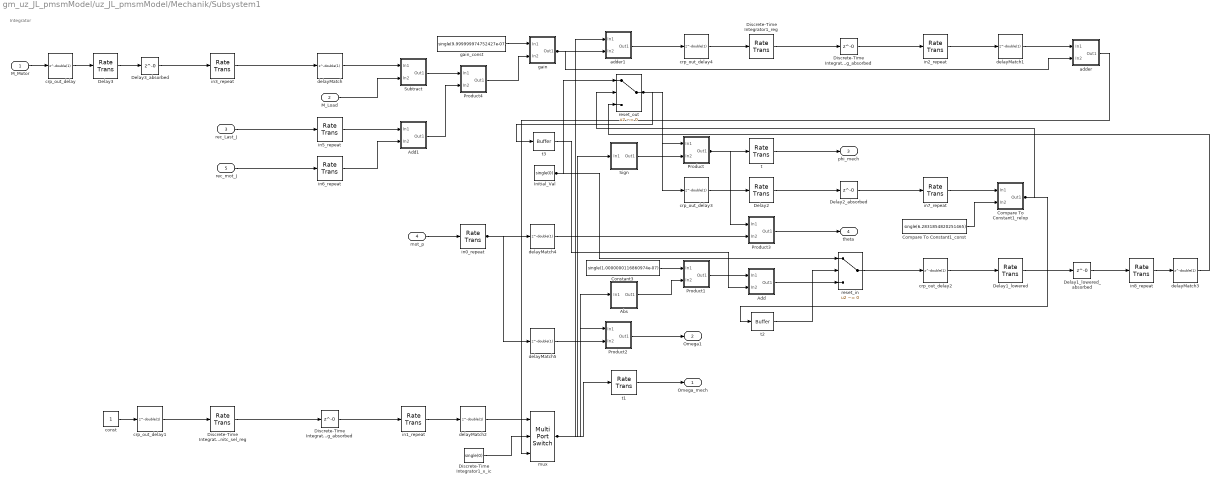
== system gm_uz_JL_pmsmModel/uz_JL_pmsmModel/Mechanik/Subsystem1 ==
  note: Integrator
  M_Motor : Inport  OutDataTypeStr=single  PortDimensions=1  SampleTime=2e-08
  M_Load : Inport  Port=2  OutDataTypeStr=single  PortDimensions=1  SampleTime=2e-08
  rec_Last_J : Inport  Port=3  OutDataTypeStr=single  PortDimensions=1  SampleTime=2e-06
  mot_p : Inport  Port=4  OutDataTypeStr=single  PortDimensions=1  SampleTime=2e-06
  rec_mot_J : Inport  Port=5  OutDataTypeStr=single  PortDimensions=1  SampleTime=2e-06
  Abs : Subsystem
      mask Display: disp('NFP\nabs');
  Add : Subsystem
      mask Display: disp('NFP\nadd');
  Add1 : Subsystem
      mask Display: disp('NFP\nadd');
  Compare To Constant1_const : Constant  Value=single(6.2831854820251465)  OutDataTypeStr=single  SampleTime=2e-08
  Compare To Constant1_relop : Subsystem
      mask Display: disp('NFP\nrelop');
  Constant3 : Constant  Value=single(1.0000000116860974e-07)  OutDataTypeStr=single  SampleTime=2e-08
  Delay1_lowered : RateTransition  InitialCondition=double(0)  OutPortSampleTimeOpt=Multiple of input port sample time  OutPortSampleTimeMultiple=100
  Delay1_lowered_absorbed : Delay  DelayLength=0
  Delay2 : RateTransition  InitialCondition=double(0)  OutPortSampleTimeOpt=Multiple of input port sample time  OutPortSampleTimeMultiple=100
  Delay2_absorbed : Delay  DelayLength=0
  Delay3 : RateTransition  InitialCondition=double(0)  OutPortSampleTimeOpt=Multiple of input port sample time  OutPortSampleTimeMultiple=100
  Delay3_absorbed : Delay  DelayLength=0
  Discrete-Time Integrator1_initc_sel_reg : RateTransition  InitialCondition=double(0)  OutPortSampleTimeOpt=Multiple of input port sample time  OutPortSampleTimeMultiple=100
  Discrete-Time Integrator1_initc_sel_reg_absorbed : Delay  DelayLength=0
  Discrete-Time Integrator1_reg : RateTransition  InitialCondition=double(0)  OutPortSampleTimeOpt=Multiple of input port sample time  OutPortSampleTimeMultiple=100
  Discrete-Time Integrator1_reg_absorbed : Delay  DelayLength=0
  Discrete-Time Integrator1_x_ic : Constant  Value=single(0)  OutDataTypeStr=single  SampleTime=2e-08
  Initial_Val : Constant  Value=single(0)  OutDataTypeStr=single  SampleTime=2e-08
  Product : Subsystem
      mask Display: disp('NFP\nmul');
  Product1 : Subsystem
      mask Display: disp('NFP\nmul');
  Product2 : Subsystem
      mask Display: disp('NFP\nmul');
  Product3 : Subsystem
      mask Display: disp('NFP\nmul');
  Product4 : Subsystem
      mask Display: disp('NFP\nmul');
  Sign : Subsystem
      mask Display: disp('NFP\nsignum');
  Subtract : Subsystem
      mask Display: disp('NFP\nadd');
  adder : Subsystem
      mask Display: disp('NFP\nadd');
  adder1 : Subsystem
      mask Display: disp('NFP\nadd');
  const : Constant  OutDataTypeStr=fixdt(0, 1, 0)  SampleTime=2e-08
  crp_out_delay{,1..4} (5 alike) : Delay  DelayLength=double(1)  InitialCondition=0  SampleTime=2e-08
  delayMatch{,1..5} (6 alike) : Delay  DelayLength=double(1)  InitialCondition=0  SampleTime=2e-08
  gain : Subsystem
      mask Display: disp('NFP\nmul');
  gain_const : Constant  Value=single(9.999999974752427e-07)  OutDataTypeStr=single  SampleTime=2e-08
  in0_repeat : RateTransition  Integrity=off  Deterministic=off  OutPortSampleTimeOpt=Multiple of input port sample time  OutPortSampleTimeMultiple=1/100
  in1_repeat : RateTransition  Integrity=off  Deterministic=off  OutPortSampleTimeOpt=Multiple of input port sample time  OutPortSampleTimeMultiple=1/100
  in2_repeat : RateTransition  Integrity=off  Deterministic=off  OutPortSampleTimeOpt=Multiple of input port sample time  OutPortSampleTimeMultiple=1/100
  in3_repeat : RateTransition  Integrity=off  Deterministic=off  OutPortSampleTimeOpt=Multiple of input port sample time  OutPortSampleTimeMultiple=1/100
  in5_repeat : RateTransition  Integrity=off  Deterministic=off  OutPortSampleTimeOpt=Multiple of input port sample time  OutPortSampleTimeMultiple=1/100
  in6_repeat : RateTransition  Integrity=off  Deterministic=off  OutPortSampleTimeOpt=Multiple of input port sample time  OutPortSampleTimeMultiple=1/100
  in7_repeat : RateTransition  Integrity=off  Deterministic=off  OutPortSampleTimeOpt=Multiple of input port sample time  OutPortSampleTimeMultiple=1/100
  in8_repeat : RateTransition  Integrity=off  Deterministic=off  OutPortSampleTimeOpt=Multiple of input port sample time  OutPortSampleTimeMultiple=1/100
  mux : MultiPortSwitch  DataPortOrder=Zero-based contiguous  Inputs=2  DiagnosticForDefault=None  zeroidx=on  OutDataTypeStr=single  SampleTime=2e-08  SaturateOnIntegerOverflow=off  InputSameDT=off
  reset_in : Switch  Criteria=u2 ~= 0  Threshold=double(0)  OutDataTypeStr=single  SampleTime=2e-08  SaturateOnIntegerOverflow=off  InputSameDT=off
  reset_out : Switch  Criteria=u2 ~= 0  Threshold=double(0)  OutDataTypeStr=single  SampleTime=2e-08  SaturateOnIntegerOverflow=off  InputSameDT=off
  t : RateTransition  InitialCondition=double(0)  OutPortSampleTimeOpt=Multiple of input port sample time  OutPortSampleTimeMultiple=100
  t1 : RateTransition  InitialCondition=double(0)  OutPortSampleTimeOpt=Multiple of input port sample time  OutPortSampleTimeMultiple=100
  t2 : hdlmdlgenlib/Buffer
  t3 : hdlmdlgenlib/Buffer
  Omega_mech : Outport  OutDataTypeStr=single  SampleTime=2e-06
  Omega1 : Outport  Port=2  OutDataTypeStr=single  SampleTime=2e-08
  phi_mech : Outport  Port=3  OutDataTypeStr=single  SampleTime=2e-06
  theta : Outport  Port=4  OutDataTypeStr=single  SampleTime=2e-08
  wires:
  delayMatch5/1 -> Product2/2(In2)
  M_Motor/1 -> crp_out_delay/1
  crp_out_delay/1 -> Delay3/1
  in3_repeat/1 -> delayMatch/1
  Delay3/1 -> Delay3_absorbed/1
  const/1 -> crp_out_delay1/1
  Subtract/1(Out1) -> Product4/1(In1)
  Delay3_absorbed/1 -> in3_repeat/1
  reset_in/1 -> crp_out_delay2/1
  delayMatch/1 -> Subtract/1(In1)
  rec_Last_J/1 -> in5_repeat/1
  crp_out_delay1/1 -> Discrete-Time Integrator1_initc_sel_reg/1
  Delay1_lowered_absorbed/1 -> in8_repeat/1
  rec_mot_J/1 -> in6_repeat/1
  in1_repeat/1 -> delayMatch2/1
  Discrete-Time Integrator1_initc_sel_reg/1 -> Discrete-Time Integrator1_initc_sel_reg_absorbed/1
  M_Load/1 -> Subtract/2(In2)
  crp_out_delay4/1 -> Discrete-Time Integrator1_reg/1
  in5_repeat/1 -> Add1/1(In1)
  in6_repeat/1 -> Add1/2(In2)
  in0_repeat/1 -> delayMatch5/1, delayMatch4/1
  Discrete-Time Integrator1_initc_sel_reg_absorbed/1 -> in1_repeat/1
  reset_out/1 -> t3/1, crp_out_delay3/1, Product/1(In1)
  Add1/1(Out1) -> Product4/2(In2)
  in8_repeat/1 -> delayMatch3/1
  mot_p/1 -> in0_repeat/1
  gain_const/1 -> gain/1(In1)
  Product4/1(Out1) -> gain/2(In2)
  delayMatch2/1 -> mux/1
  Product/1(Out1) -> t/1, Product3/1(In1)
  Discrete-Time Integrator1_x_ic/1 -> mux/2
  gain/1(Out1) -> adder/2(In2), adder1/2(In2)
  t3/1 -> Add/2(In2)
  delayMatch3/1 -> reset_out/3
  Initial_Val/1 -> reset_in/1, reset_out/1
  delayMatch4/1 -> Product3/2(In2)
  Delay2/1 -> Delay2_absorbed/1
  mux/1 -> Sign/1(In1), Abs/1(In1), Product2/1(In1), adder1/1(In1), t1/1
  adder1/1(Out1) -> crp_out_delay4/1
  Sign/1(Out1) -> Product/2(In2)
  Constant3/1 -> Product1/1(In1)
  Abs/1(Out1) -> Product1/2(In2)
  Product2/1(Out1) -> Omega1/1
  adder/1(Out1) -> mux/3
  t1/1 -> Omega_mech/1
  crp_out_delay3/1 -> Delay2/1
  Product1/1(Out1) -> Add/1(In1)
  Discrete-Time Integrator1_reg/1 -> Discrete-Time Integrator1_reg_absorbed/1
  t/1 -> phi_mech/1
  crp_out_delay2/1 -> Delay1_lowered/1
  Product3/1(Out1) -> theta/1
  Add/1(Out1) -> reset_in/3
  t2/1 -> reset_in/2
  Compare To Constant1_relop/1(Out1) -> t2/1, reset_out/2
  Compare To Constant1_const/1 -> Compare To Constant1_relop/2(In2)
  Discrete-Time Integrator1_reg_absorbed/1 -> in2_repeat/1
  Delay2_absorbed/1 -> in7_repeat/1
  in2_repeat/1 -> delayMatch1/1
  in7_repeat/1 -> Compare To Constant1_relop/1(In1)
  delayMatch1/1 -> adder/1(In1)
  Delay1_lowered/1 -> Delay1_lowered_absorbed/1

== system gm_uz_JL_pmsmModel/uz_JL_pmsmModel/Elektrik/Psi/Product1 ==
  In1 : Inport
  In2 : Inport  Port=2
  Product1 : Product  Inputs=**  OutDataTypeStr=single  SampleTime=2e-08
  Product1_pd1 : Delay  DelayLength=6
  Out1 : Outport
  wires:
  In1/1 -> Product1/1
  In2/1 -> Product1/2
  Product1/1 -> Product1_pd1/1
  Product1_pd1/1 -> Out1/1

== system gm_uz_JL_pmsmModel/uz_JL_pmsmModel/Elektrik/Psi/Product2 ==
  In1 : Inport
  In2 : Inport  Port=2
  Product2 : Product  Inputs=**  OutDataTypeStr=single  SampleTime=2e-08
  Product2_pd1 : Delay  DelayLength=6
  Out1 : Outport
  wires:
  In1/1 -> Product2/1
  In2/1 -> Product2/2
  Product2/1 -> Product2_pd1/1
  Product2_pd1/1 -> Out1/1

== system gm_uz_JL_pmsmModel/uz_JL_pmsmModel/Elektrik/Psi/Product3 ==
  In1 : Inport
  In2 : Inport  Port=2
  Product3 : Product  Inputs=**  OutDataTypeStr=single  SampleTime=2e-08
  Product3_pd1 : Delay  DelayLength=6
  Out1 : Outport
  wires:
  In1/1 -> Product3/1
  In2/1 -> Product3/2
  Product3/1 -> Product3_pd1/1
  Product3_pd1/1 -> Out1/1

== system gm_uz_JL_pmsmModel/uz_JL_pmsmModel/Elektrik/Psi/Product4 ==
  In1 : Inport
  In2 : Inport  Port=2
  Product4 : Product  Inputs=**  OutDataTypeStr=single  SampleTime=2e-08
  Product4_pd1 : Delay  DelayLength=6
  Out1 : Outport
  wires:
  In1/1 -> Product4/1
  In2/1 -> Product4/2
  Product4/1 -> Product4_pd1/1
  Product4_pd1/1 -> Out1/1

== system gm_uz_JL_pmsmModel/uz_JL_pmsmModel/Elektrik/Psi/Subtract2_stage2 ==
  In1 : Inport
  In2 : Inport  Port=2
  Subtract2_stage2 : Sum  OutDataTypeStr=single  SampleTime=2e-08
  Subtract2_stage2_pd1 : Delay  DelayLength=6
  Out1 : Outport
  wires:
  In1/1 -> Subtract2_stage2/1
  In2/1 -> Subtract2_stage2/2
  Subtract2_stage2/1 -> Subtract2_stage2_pd1/1
  Subtract2_stage2_pd1/1 -> Out1/1

== system gm_uz_JL_pmsmModel/uz_JL_pmsmModel/Elektrik/Psi/Subtract2_stage3 ==
  In1 : Inport
  In2 : Inport  Port=2
  Subtract2_stage3 : Sum  Inputs=+-  OutDataTypeStr=single  SampleTime=2e-08
  Subtract2_stage3_pd1 : Delay  DelayLength=6
  Out1 : Outport
  wires:
  In1/1 -> Subtract2_stage3/1
  In2/1 -> Subtract2_stage3/2
  Subtract2_stage3/1 -> Subtract2_stage3_pd1/1
  Subtract2_stage3_pd1/1 -> Out1/1

== system gm_uz_JL_pmsmModel/uz_JL_pmsmModel/Elektrik/Psi/Subtract3_stage2 ==
  In1 : Inport
  In2 : Inport  Port=2
  Subtract3_stage2 : Sum  Inputs=+-  OutDataTypeStr=single  SampleTime=2e-08
  Subtract3_stage2_pd1 : Delay  DelayLength=6
  Out1 : Outport
  wires:
  In1/1 -> Subtract3_stage2/1
  In2/1 -> Subtract3_stage2/2
  Subtract3_stage2/1 -> Subtract3_stage2_pd1/1
  Subtract3_stage2_pd1/1 -> Out1/1

== system gm_uz_JL_pmsmModel/uz_JL_pmsmModel/Elektrik/Psi/Subtract3_stage3 ==
  In1 : Inport
  In2 : Inport  Port=2
  Subtract3_stage3 : Sum  Inputs=+-  OutDataTypeStr=single  SampleTime=2e-08
  Subtract3_stage3_pd1 : Delay  DelayLength=6
  Out1 : Outport
  wires:
  In1/1 -> Subtract3_stage3/1
  In2/1 -> Subtract3_stage3/2
  Subtract3_stage3/1 -> Subtract3_stage3_pd1/1
  Subtract3_stage3_pd1/1 -> Out1/1

== system gm_uz_JL_pmsmModel/uz_JL_pmsmModel/Elektrik/Psi/Sum ==
  In1 : Inport
  In2 : Inport  Port=2
  Sum : Sum  OutDataTypeStr=single  SampleTime=2e-08
  Sum_pd1 : Delay  DelayLength=6
  Out1 : Outport
  wires:
  In1/1 -> Sum/1
  In2/1 -> Sum/2
  Sum/1 -> Sum_pd1/1
  Sum_pd1/1 -> Out1/1

== system gm_uz_JL_pmsmModel/uz_JL_pmsmModel/Elektrik/Psi/adder ==
  In1 : Inport
  In2 : Inport  Port=2
  adder : Sum  OutDataTypeStr=single  SampleTime=2e-08
  adder_pd1 : Delay  DelayLength=6
  Out1 : Outport
  wires:
  In1/1 -> adder/1
  In2/1 -> adder/2
  adder/1 -> adder_pd1/1
  adder_pd1/1 -> Out1/1

== system gm_uz_JL_pmsmModel/uz_JL_pmsmModel/Elektrik/Psi/adder1 ==
  In1 : Inport
  In2 : Inport  Port=2
  adder1 : Sum  OutDataTypeStr=single  SampleTime=2e-08
  adder1_pd1 : Delay  DelayLength=6
  Out1 : Outport
  wires:
  In1/1 -> adder1/1
  In2/1 -> adder1/2
  adder1/1 -> adder1_pd1/1
  adder1_pd1/1 -> Out1/1

== system gm_uz_JL_pmsmModel/uz_JL_pmsmModel/Elektrik/Psi/gain ==
  In1 : Inport
  In2 : Inport  Port=2
  gain : Product  Inputs=**  OutDataTypeStr=single  SampleTime=2e-08
  gain_pd1 : Delay  DelayLength=6
  Out1 : Outport
  wires:
  In1/1 -> gain/1
  In2/1 -> gain/2
  gain/1 -> gain_pd1/1
  gain_pd1/1 -> Out1/1

== system gm_uz_JL_pmsmModel/uz_JL_pmsmModel/Elektrik/Psi/gain1 ==
  In1 : Inport
  In2 : Inport  Port=2
  gain1 : Product  Inputs=**  OutDataTypeStr=single  SampleTime=2e-08
  gain1_pd1 : Delay  DelayLength=6
  Out1 : Outport
  wires:
  In1/1 -> gain1/1
  In2/1 -> gain1/2
  gain1/1 -> gain1_pd1/1
  gain1_pd1/1 -> Out1/1

== system gm_uz_JL_pmsmModel/uz_JL_pmsmModel/Elektrik/Subsystem2/Product ==
  In1 : Inport
  In2 : Inport  Port=2
  Product : Product  Inputs=**  OutDataTypeStr=single  SampleTime=2e-08
  Product_pd1 : Delay  DelayLength=6
  Out1 : Outport
  wires:
  In1/1 -> Product/1
  In2/1 -> Product/2
  Product/1 -> Product_pd1/1
  Product_pd1/1 -> Out1/1

== system gm_uz_JL_pmsmModel/uz_JL_pmsmModel/Elektrik/Subsystem2/Product1 ==
  In1 : Inport
  In2 : Inport  Port=2
  Product1 : Product  Inputs=**  OutDataTypeStr=single  SampleTime=2e-08
  Product1_pd1 : Delay  DelayLength=6
  Out1 : Outport
  wires:
  In1/1 -> Product1/1
  In2/1 -> Product1/2
  Product1/1 -> Product1_pd1/1
  Product1_pd1/1 -> Out1/1

== system gm_uz_JL_pmsmModel/uz_JL_pmsmModel/Elektrik/Subsystem2/Subtract ==
  In1 : Inport
  In2 : Inport  Port=2
  Subtract : Sum  Inputs=+-  OutDataTypeStr=single  SampleTime=2e-08
  Subtract_pd1 : Delay  DelayLength=6
  Out1 : Outport
  wires:
  In1/1 -> Subtract/1
  In2/1 -> Subtract/2
  Subtract/1 -> Subtract_pd1/1
  Subtract_pd1/1 -> Out1/1

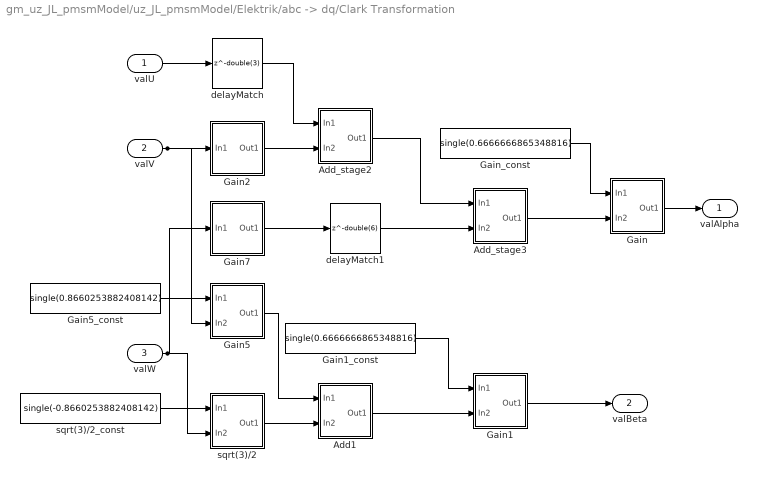
== system gm_uz_JL_pmsmModel/uz_JL_pmsmModel/Elektrik/abc -> dq/Clark Transformation ==
  valU : Inport  OutDataTypeStr=single  PortDimensions=1  SampleTime=2e-08
  valV : Inport  Port=2  OutDataTypeStr=single  PortDimensions=1  SampleTime=2e-08
  valW : Inport  Port=3  OutDataTypeStr=single  PortDimensions=1  SampleTime=2e-08
  Add1 : Subsystem
      mask Display: disp('NFP\nadd');
  Add_stage2 : Subsystem
      mask Display: disp('NFP\nadd');
  Add_stage3 : Subsystem
      mask Display: disp('NFP\nadd');
  Gain : Subsystem
      mask Display: disp('NFP\nmul');
  Gain1 : Subsystem
      mask Display: disp('NFP\nmul');
  Gain1_const : Constant  Value=single(0.6666666865348816)  OutDataTypeStr=single  SampleTime=2e-08
  Gain2 : Subsystem
      mask Display: disp('NFP\ngain_pow2');
  Gain5 : Subsystem
      mask Display: disp('NFP\nmul');
  Gain5_const : Constant  Value=single(0.8660253882408142)  OutDataTypeStr=single  SampleTime=2e-08
  Gain7 : Subsystem
      mask Display: disp('NFP\ngain_pow2');
  Gain_const : Constant  Value=single(0.6666666865348816)  OutDataTypeStr=single  SampleTime=2e-08
  delayMatch : Delay  DelayLength=double(3)  InitialCondition=0  SampleTime=2e-08
  delayMatch1 : Delay  DelayLength=double(6)  InitialCondition=0  SampleTime=2e-08
  sqrt(3)/2 : Subsystem
      mask Display: disp('NFP\nmul');
  sqrt(3)/2_const : Constant  Value=single(-0.8660253882408142)  OutDataTypeStr=single  SampleTime=2e-08
  valAlpha : Outport  SampleTime=2e-08
  valBeta : Outport  Port=2  SampleTime=2e-08
  wires:
  valU/1 -> delayMatch/1
  Gain5_const/1 -> Gain5/1(In1)
  valV/1 -> Gain5/2(In2), Gain2/1(In1)
  valW/1 -> Gain7/1(In1), sqrt(3)/2/2(In2)
  delayMatch/1 -> Add_stage2/1(In1)
  sqrt(3)/2_const/1 -> sqrt(3)/2/1(In1)
  Gain2/1(Out1) -> Add_stage2/2(In2)
  Gain7/1(Out1) -> delayMatch1/1
  Gain5/1(Out1) -> Add1/1(In1)
  sqrt(3)/2/1(Out1) -> Add1/2(In2)
  Add_stage2/1(Out1) -> Add_stage3/1(In1)
  delayMatch1/1 -> Add_stage3/2(In2)
  Gain1_const/1 -> Gain1/1(In1)
  Add1/1(Out1) -> Gain1/2(In2)
  Gain_const/1 -> Gain/1(In1)
  Add_stage3/1(Out1) -> Gain/2(In2)
  Gain1/1(Out1) -> valBeta/1
  Gain/1(Out1) -> valAlpha/1
